simulink model "Rover_Simulation"  (R2023b)
settings: Solver=VariableStepAuto  StartTime=0.0  StopTime=10.0  RelTol=1e-3
values from neighbouring files (symbols this model uses):
  q0 = zeros(3,1)    [Initialisierung_Rover_.m]
undefined symbols (not defined in the file or in its folder): roverLength, roverWidth, wheelRadius
settings Model: Creator=Asus  LastModifiedBy=sth0064
settings RTWCC: GPUComputeCapability=5.0

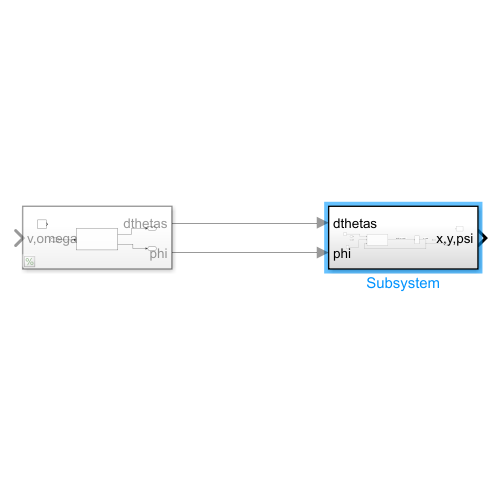
[thumbnail: Simulink's stored preview of the top-level diagram]
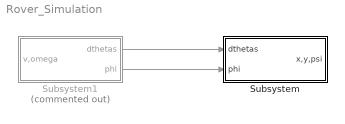
== system Rover_Simulation ==
  Subsystem : Subsystem
  Subsystem1 : Subsystem  Commented=on
  wires:
  Subsystem1/1(dthetas) -> Subsystem/1(dthetas)
  Subsystem1/2(phi) -> Subsystem/2(phi)

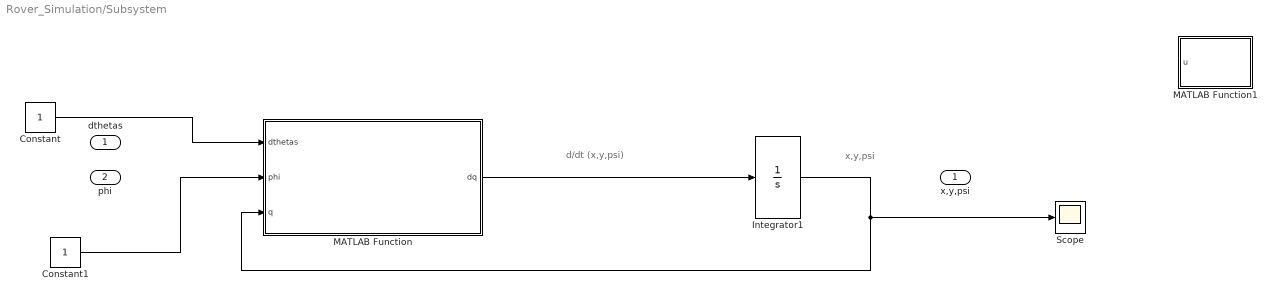
== system Rover_Simulation/Subsystem ==
  note: d/dt (x,y,psi)
  note: x,y,psi
  dthetas : Inport
  phi : Inport  Port=2
  Constant : Constant
  Constant1 : Constant
  Integrator1 : Integrator  InitialCondition=q0
  MATLAB Function : MATLAB Function  TreatAsAtomicUnit=on
  MATLAB Function1 : MATLAB Function  TreatAsAtomicUnit=on
  Scope : Scope
  x,y,psi : Outport
  wires:
  Constant/1 -> MATLAB Function/1(dthetas)
  MATLAB Function/1(dq) -> Integrator1/1
  Integrator1/1 -> MATLAB Function/3(q), Scope/1
  Constant1/1 -> MATLAB Function/2(phi)

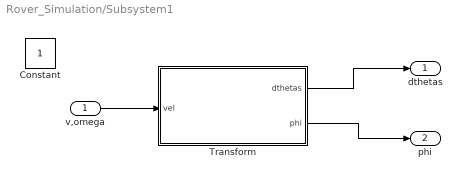
== system Rover_Simulation/Subsystem1 ==
  v,omega : Inport
  Constant : Constant
  Transform : MATLAB Function  TreatAsAtomicUnit=on
  dthetas : Outport
  phi : Outport  Port=2
  wires:
  Transform/2(phi) -> phi/1
  v,omega/1 -> Transform/1(vel)
  Transform/1(dthetas) -> dthetas/1

== matlab function Rover_Simulation/Subsystem1/Transform ==
  data: vel input; dthetas output; phi output; roverWidth parameter; wheelRadius parameter; roverLength parameter
function [dthetas, phi] = fcn(vel, roverWidth, wheelRadius, roverLength)


dtheta1 = (1/wheelRadius)*sqrt((vel(1) + 0.5*vel(2)*roverWidth)^2 + (0.5*vel(2)*roverLength)^2);
dtheta2 = (1/wheelRadius)*sqrt((vel(1) - 0.5*vel(2)*roverWidth)^2 + (0.5*vel(2)*roverLength)^2);
dtheta3 = (1/wheelRadius)*sqrt((vel(1) - 0.5*vel(2)*roverWidth)^2 + (-0.5*vel(2)*roverLength)^2);
dtheta4 = (1/wheelRadius)*sqrt((vel(1) + 0.5*vel(2)*roverWidth)^2 + (-0.5*vel(2)*roverLength)^2);


phi1 = atan(0.5 * vel(2) * roverLength / (vel(1) + 0.5*vel(2)*roverWidth));
phi2 = atan(0.5 * vel(2) * roverLength / (vel(1) - 0.5*vel(2)*roverWidth));
phi3 = atan(-0.5 * vel(2) * roverLength / (vel(1) - 0.5*vel(2)*roverWidth));
phi4 = atan(-0.5 * vel(2) * roverLength / (vel(1) + 0.5*vel(2)*roverWidth));

dthetas = [dtheta1, dtheta2, dtheta3, dtheta4];
phi = [phi1, phi2, phi3, phi4];

end

== matlab function Rover_Simulation/Subsystem/MATLAB Function1 ==
  data: u input
function plot_vehicle(u)
%#codegen
coder.extrinsic('fct_plot_vehicle')

x = u(1);
y = u(2);
psi = u(3);

fct_plot_vehicle(x, y);
end

== matlab function Rover_Simulation/Subsystem/MATLAB Function ==
  data: dthetas input; phi input; q input; dq output; wheelRadius parameter; roverWidth parameter
function dq = fcn(dthetas, phi, q, wheelRadius, roverWidth)

% wenn wheelRadius kein input ist, kommt es dann aus der Workspace?

psi = q(3); 

dq = zeros(3,1);

q0 = zeros(3,1);

% Rotationsmatrix
Rz = [cos(psi) -sin(psi) 0;
    sin(psi) cos(psi) 0;
    0 0 1];

% Lokale Geschwindigkeiten
vx = (wheelRadius/4) * (dthetas(1)*cos(phi(1)) + dthetas(2)*cos(phi(2)) + ...
                        dthetas(3)*cos(phi(3)) + dthetas(4)*cos(phi(4))); 

vy = (wheelRadius/4) * (dthetas(1)*sin(phi(1)) + dthetas(2)*sin(phi(2)) + ...
                        dthetas(3)*sin(phi(3)) + dthetas(4)*sin(phi(4)));

omega = (wheelRadius/2*roverWidth) * (dthetas(1)*cos(phi(1)) - dthetas(2)*cos(phi(2)) - ...
                        dthetas(3)*cos(phi(3)) + dthetas(4)*cos(phi(4)));

roverSpeedLoc = [vx vy omega]';

dq = Rz*roverSpeedLoc;
